simulink model "Board_Case_1"  (R2018b)
settings: Solver=FixedStepAuto  StartTime=0.0  StopTime=1000  FixedStep=0.01  RelTol=1e-3  EnableMultiTasking=on
libraries: simulink x4, svdutilitieslib x2, arduinolib x2
settings Model: ExtModeTrigDuration=2  Creator=AmiR_KhaN  LastModifiedBy=User
settings OptimizationCC: EnhancedBackFolding=on  PassReuseOutputArgsAs=Individual arguments  MaxStackSize=64  OptimizeBlockOrder=speed  DifferentSizesBufferReuse=on  OptimizationCustomize=off
settings DebuggingCC: ParameterTunabilityLossMsg=error
settings HardwareCC: ProdBitPerInt=16  ProdBitPerPointer=16  ProdBitPerSizeT=16  ProdBitPerPtrDiffT=16  ProdLargestAtomicFloat=None  ProdWordSize=8  ProdHWDeviceType=Atmel->AVR
settings SFSimCC: MATLABDynamicMemAlloc=off
settings RTWCC: SystemTargetFile=ert.tlc  HardwareBoard=Arduino Uno  TemplateMakefile=ert_default_tmf  GenerateReport=on  Toolchain=Arduino AVR  BuildConfiguration=Faster Runs  IncludeHyperlinkInReport=on  LaunchReport=on  GenerateTraceInfo=on  GenerateTraceReport=on  GenerateTraceReportSl=on  GenerateTraceReportSf=on  GenerateTraceReportEml=on
settings CodeAppCC: ForceParamTrailComments=on  IgnoreCustomStorageClasses=off  OperatorAnnotations=on  SimulinkDataObjDesc=on  SFDataObjDesc=on  InsertBlockDesc=on
settings ERTTargetCC: SupportContinuousTime=on  SupportVariableSizeSignals=on  ExtModeStaticAllocSize=250

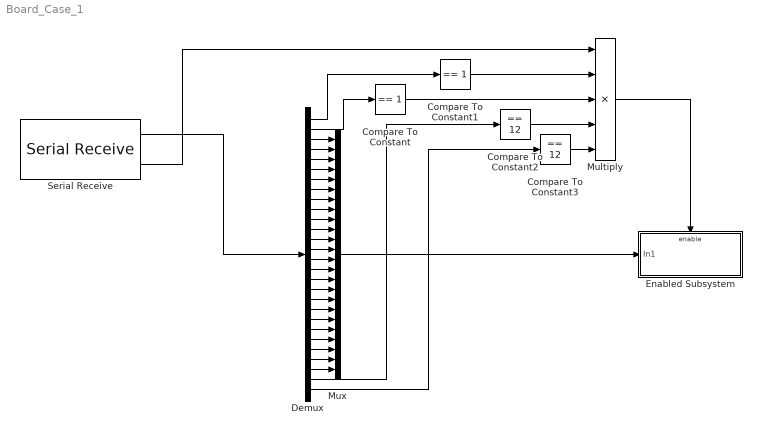
== system Board_Case_1 ==
  Compare To Constant : simulink/Logic and Bit Operations/Compare To Constant  relop===  const=1  OutDataTypeStr=boolean
  Compare To Constant1 : simulink/Logic and Bit Operations/Compare To Constant  relop===  const=1  OutDataTypeStr=boolean
  Compare To Constant2 : simulink/Logic and Bit Operations/Compare To Constant  relop===  const=12  OutDataTypeStr=boolean
  Compare To Constant3 : simulink/Logic and Bit Operations/Compare To Constant  relop===  const=12  OutDataTypeStr=boolean
  Demux : Demux  Outputs=28
  Enabled Subsystem : Subsystem  TreatAsAtomicUnit=on
  Multiply : Product  Inputs=5
  Mux : Mux  Inputs=24
  Serial Receive : arduinolib/Serial Receive  isARMArch=off  portNumber=0  DataType=uint8  Datalength=28  SampleTime=0.01  showOutStatus=on  blockPlatform=arduino
      settings: SourceProductBaseCode=ARDUINO
  wires:
  Multiply/1 -> Enabled Subsystem/Enable
  Compare To Constant2/1 -> Multiply/4
  Mux/1 -> Enabled Subsystem/1(In1)
  Compare To Constant3/1 -> Multiply/5
  Serial Receive/2 -> Multiply/1
  Serial Receive/1 -> Demux/1
  Demux/1 -> Compare To Constant1/1
  Demux/2 -> Compare To Constant/1
  Compare To Constant1/1 -> Multiply/2
  Compare To Constant/1 -> Multiply/3
  Demux/28 -> Compare To Constant3/1
  Demux/27 -> Compare To Constant2/1
  Demux/3 -> Mux/1
  Demux/4 -> Mux/2
  Demux/5 -> Mux/3
  Demux/6 -> Mux/4
  Demux/7 -> Mux/5
  Demux/8 -> Mux/6
  Demux/9 -> Mux/7
  Demux/10 -> Mux/8
  Demux/11 -> Mux/9
  Demux/12 -> Mux/10
  Demux/13 -> Mux/11
  Demux/14 -> Mux/12
  Demux/15 -> Mux/13
  Demux/16 -> Mux/14
  Demux/17 -> Mux/15
  Demux/18 -> Mux/16
  Demux/19 -> Mux/17
  Demux/20 -> Mux/18
  Demux/21 -> Mux/19
  Demux/22 -> Mux/20
  Demux/23 -> Mux/21
  Demux/24 -> Mux/22
  Demux/25 -> Mux/23
  Demux/26 -> Mux/24

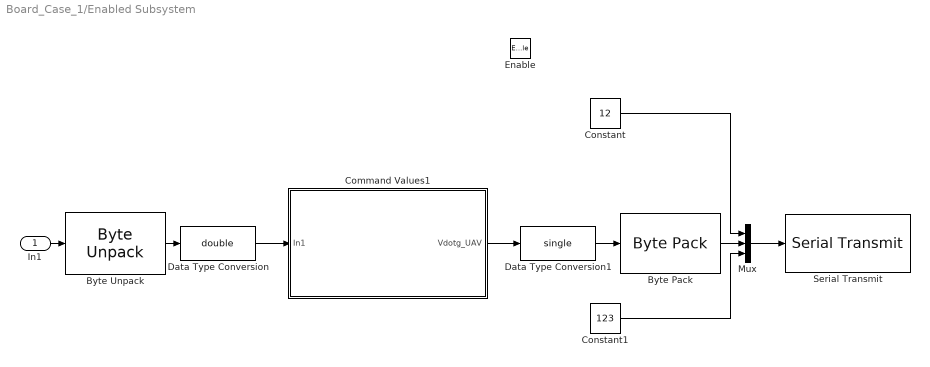
== system Board_Case_1/Enabled Subsystem ==
  In1 : Inport
  Enable : EnablePort
  Byte Pack : svdutilitieslib/Byte Pack  maskPackedDataType=uint8  datatypes={'single'}  byteAlign=4  blockPlatform=arduinoert
      settings: SourceProductBaseCode=ARDUINO,ML_ARDUINO,ECCORTEXA,ECCORTEXR,SC_BEAGLEBONE_BLUE,EC_FREEDOM_BOARD,EC_FRDM_K64F,INTEL_BLOCKSET,MICROBIT,NUCLEO,PX4AUTOPILOTS,RASPPIIO,STMICRODIS,TIC2000,XILINX_BLOCKSET
  Byte Unpack : svdutilitieslib/Byte Unpack  dimensions={[6]}  datatypes={'single'}  byteAlign=4  blockPlatform=arduinoert
      settings: SourceProductBaseCode=ARDUINO,ML_ARDUINO,ECCORTEXA,ECCORTEXR,SC_BEAGLEBONE_BLUE,EC_FREEDOM_BOARD,EC_FRDM_K64F,INTEL_BLOCKSET,MICROBIT,NUCLEO,PX4AUTOPILOTS,RASPPIIO,STMICRODIS,TIC2000,XILINX_BLOCKSET
  Command Values1 : Subsystem
  Constant : Constant  Value=12  OutDataTypeStr=uint8
  Constant1 : Constant  Value=123  OutDataTypeStr=uint8
  Data Type Conversion : DataTypeConversion  OutDataTypeStr=double
  Data Type Conversion1 : DataTypeConversion  OutDataTypeStr=single
  Mux : Mux  Inputs=3
  Serial Transmit : arduinolib/Serial Transmit  portNumber=0  sendmode=write  sendformat=Decimal  floatprecision=2  blockPlatform=arduino
  wires:
  Command Values1/1(Vdotg_UAV) -> Data Type Conversion1/1
  In1/1 -> Byte Unpack/1
  Byte Unpack/1 -> Data Type Conversion/1
  Data Type Conversion/1 -> Command Values1/1(In1)
  Data Type Conversion1/1 -> Byte Pack/1
  Byte Pack/1 -> Mux/2
  Constant/1 -> Mux/1
  Constant1/1 -> Mux/3
  Mux/1 -> Serial Transmit/1

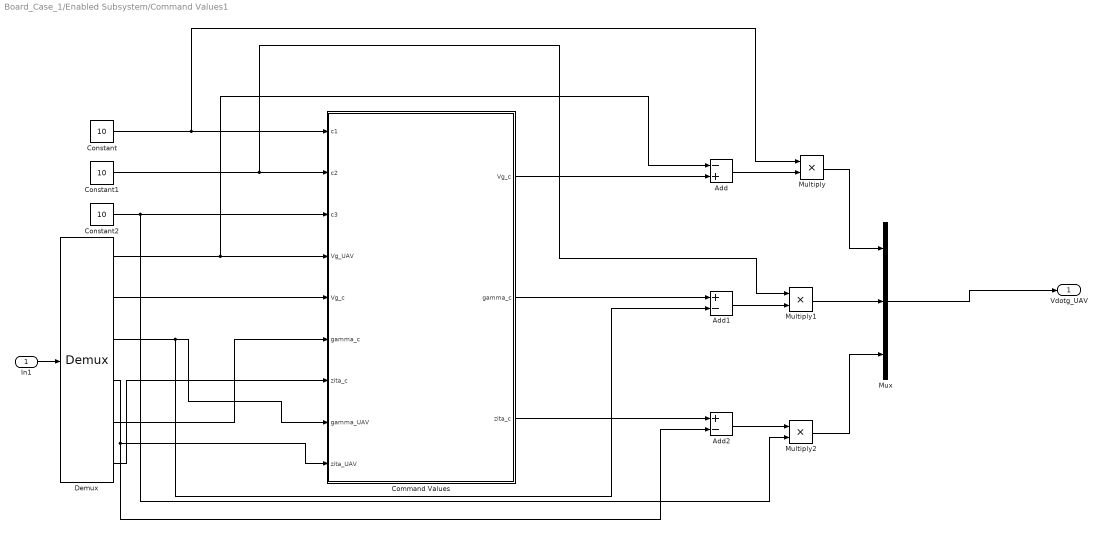
== system Board_Case_1/Enabled Subsystem/Command Values1 ==
  In1 : Inport
  Add : Sum  Inputs=-+
  Add1 : Sum  Inputs=+-
  Add2 : Sum  Inputs=+-
  Command Values : MATLAB Function  TreatAsAtomicUnit=on
  Constant : Constant  Value=10
  Constant1 : Constant  Value=10
  Constant2 : Constant  Value=10
  Demux : Demux  Outputs=6
  Multiply : Product
  Multiply1 : Product
  Multiply2 : Product
  Mux : Mux  Inputs=3
  Vdotg_UAV : Outport
  wires:
  Command Values/2(gamma_c) -> Add1/1
  Command Values/3(zita_c) -> Add2/1
  Demux/1 -> Add/1, Command Values/4(Vg_UAV)
  Demux/2 -> Command Values/5("Vg_c ")
  Constant/1 -> Multiply/1, Command Values/1(c1)
  Constant1/1 -> Multiply1/1, Command Values/2(c2)
  Constant2/1 -> Command Values/3(c3), Multiply2/2
  Command Values/1(Vg_c) -> Add/2
  Add/1 -> Multiply/2
  Add1/1 -> Multiply1/2
  Add2/1 -> Multiply2/1
  In1/1 -> Demux/1
  Demux/5 -> Command Values/6("gamma_c ")
  Demux/6 -> Command Values/7("zita_c ")
  Demux/3 -> Add1/2, Command Values/8(gamma_UAV)
  Demux/4 -> Add2/2, Command Values/9(zita_UAV)
  Multiply/1 -> Mux/1
  Multiply1/1 -> Mux/2
  Multiply2/1 -> Mux/3
  Mux/1 -> Vdotg_UAV/1

== matlab function Board_Case_1/Enabled Subsystem/Command Values1/Command Values ==
  data: c1 input; Vg_c output; c2 input; c3 input; Vg_UAV input; Vg_c input; gamma_c input; zita_c input; gamma_c output; zita_c output; gamma_UAV input; zita_UAV input
function [Vg_c,gamma_c,zita_c] = fcn(c1,c2,c3,Vg_UAV,Vg_c,gamma_c,zita_c,gamma_UAV,zita_UAV)

Vg_c = Vg_UAV - (1/c1)*(Vg_c);
gamma_c = gamma_UAV - (1/(c2*Vg_UAV))*(gamma_c);
zita_c = zita_UAV - (1/c3)*zita_c;
